simulink model "poredjenje_regulatora_nelinearni_model"  (R2018a)
settings: Solver=ode4  StartTime=0.0  StopTime=150  FixedStep=0.01  RelTol=1e-3  EnableMultiTasking=on
values from neighbouring files (symbols this model uses):
  a1 = K_dek(1, 1)    [skript_drugi_deo.m]
  a2 = K_dek(1, 2)    [skript_drugi_deo.m]
  a3 = K_dek(2, 1)    [skript_drugi_deo.m]
  a4 = K_dek(2, 2)    [skript_drugi_deo.m]
  Ar1 = 0.04    [skript_drugi_deo.m]
  Ar2 = 0.04    [skript_drugi_deo.m]
  Cd1 = 0.65    [skript_drugi_deo.m]
  Cd2 = 0.65    [skript_drugi_deo.m]
  Cdh = 0.65    [skript_drugi_deo.m]
  dT = 0.1    [skript_drugi_deo.m]
  g = 9.81    [skript_drugi_deo.m]
  H1_max = 1.5    [skript_drugi_deo.m]
  H1_min = 0    [skript_drugi_deo.m]
  H1_N = 0.7    [skript_drugi_deo.m]
  H2_max = 1.5    [skript_drugi_deo.m]
  H2_min = 0    [skript_drugi_deo.m]
  H2_N = 0.8    [skript_drugi_deo.m]
  Kv1 = 1.5/1000    (= 0.0015)    [skript_drugi_deo.m]
  Kv2 = 1.5/1000    (= 0.0015)    [skript_drugi_deo.m]
  Kvh = 1/1000    (= 0.001)    [skript_drugi_deo.m]
  Ph = 3.25*10^5    (= 325000)    [skript_drugi_deo.m]
  ro = 1000    [skript_drugi_deo.m]
  Uv1 = 3    [skript_drugi_deo.m]
  Uv2_max = 10    [skript_drugi_deo.m]
  Uv2_min = 0    [skript_drugi_deo.m]
  Uv2_N = double(solve(e2 == 0, U2_N))    [skript_drugi_deo.m]
  Uvh_max = 10    [skript_drugi_deo.m]
  Uvh_min = 0    [skript_drugi_deo.m]
  Uvh_N = double(solve(e1 == 0, Uh_N))    [skript_drugi_deo.m]
  w1 = 0.1    [skript_drugi_deo.m]
  w2 = 0.1    [skript_drugi_deo.m]
  wh = 0.03    [skript_drugi_deo.m]
undefined symbols (not defined in the file or in its folder): den_d1, den_d2, num_d1, num_d2
libraries: simulink x2
settings Model: Creator=Nikola  LastModifiedBy=lakim
settings DataIOCC: LimitDataPoints=on  SaveFormat=Array
settings OptimizationCC: LifeSpan=inf
settings DebuggingCC: SFUnexpectedBacktrackingDiag=warning  SFNoUnconditionalDefaultTransitionDiag=warning  SFExecutionAtInitializationDiag=none
settings HardwareCC: ProdBitPerPointer=32  ProdBitPerSizeT=32  ProdBitPerPtrDiffT=32  ProdLargestAtomicFloat=None  ProdIntDivRoundTo=Undefined  ProdEndianess=Unspecified  ProdWordSize=32  ProdHWDeviceType=32-bit Generic
settings ModelReferenceCC: PropagateSignalLabelsOutOfModel=off
settings CodeAppCC: StateflowObjectComments=on
settings GRTTargetCC: TargetLangStandard=C89/C90 (ANSI)  GeneratePreprocessorConditionals=Disable all
settings ConfigComp: CovMetricSettings=dw  CovHtmlReporting=on  CovSaveCumulativeToWorkspaceVar=on  CovSaveSingleToWorkspaceVar=on  CovExternalEMLEnable=off

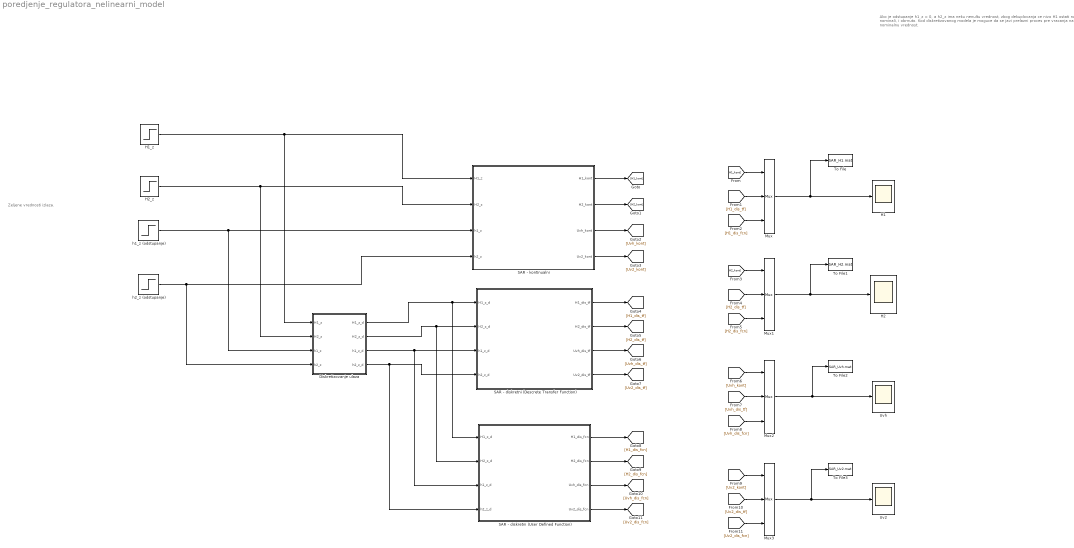
== system poredjenje_regulatora_nelinearni_model ==
  note: Ako je odstupanje h1_z = 0, a h2_z ima neku nenultu vrednost,
      | zbog dekuplovanja ce nivo H1 ostati na nominali, i obrnuto.
      | Kod diskretizovanog modela je moguce da se javi prelazni
      | proces pre vracanja na nominalnu vrednost.
  note: Zeljene vrednosti izlaza.
  Diskretizovanje ulaza : Subsystem
  H1 : Scope
  "H1_z " : Step  Time=0  After=H1_N  SampleTime=0
  H2 : Scope
  H2_z : Step  Time=0  After=H2_N  SampleTime=0
  Mux{,1..3} (4 alike) : Mux  Inputs=3
  SAR - diskretni (Descrete Transfer Function) : Subsystem
  SAR - diskretni (User Defined Function) : Subsystem
  SAR - kontinualni : Subsystem
  To File : ToFile  Filename=SAR_H1.mat  MatrixName=H1_r
  To File1 : ToFile  Filename=SAR_H2.mat  MatrixName=H2_r
  To File2 : ToFile  Filename=SAR_Uvh.mat  MatrixName=Uvh_r
  To File3 : ToFile  Filename=SAR_Uv2.mat  MatrixName=Uv2_r
  "Uv2 " : Scope
  "Uvh  " : Scope
  h1_z (odstupanje) : Step  Time=0  After=0.1  SampleTime=0
  h2_z (odstupanje) : Step  Time=0  After=0  SampleTime=0
  wires:
  "H1_z "/1 -> Diskretizovanje ulaza/1(H1_z), SAR - kontinualni/1(H1_z)
  H2_z/1 -> Diskretizovanje ulaza/2(H2_z), SAR - kontinualni/2(H2_z)
  h1_z (odstupanje)/1 -> Diskretizovanje ulaza/3(h1_z), SAR - kontinualni/3(h1_z)
  h2_z (odstupanje)/1 -> Diskretizovanje ulaza/4(h2_z), SAR - kontinualni/4(h2_z)
  Diskretizovanje ulaza/1(H1_z_d) -> SAR - diskretni (User Defined Function)/1(H1_z_d), SAR - diskretni (Descrete Transfer Function)/1(H1_z_d)
  Diskretizovanje ulaza/2(H2_z_d) -> SAR - diskretni (User Defined Function)/2(H2_z_d), SAR - diskretni (Descrete Transfer Function)/2(H2_z_d)
  Diskretizovanje ulaza/3(h1_z_d) -> SAR - diskretni (User Defined Function)/3(h1_z_d), SAR - diskretni (Descrete Transfer Function)/3(h1_z_d)
  Diskretizovanje ulaza/4(h2_z_d) -> SAR - diskretni (User Defined Function)/4(h2_z_d), SAR - diskretni (Descrete Transfer Function)/4(h2_z_d)
  Mux/1 -> To File/1, H1/1
  Mux1/1 -> To File1/1, H2/1
  SAR - kontinualni/1(H1_kont) -> [H1_kont]
  SAR - kontinualni/2(H2_kont) -> [H2_kont]
  SAR - kontinualni/3(Uvh_kont) -> [Uvh_kont]
  SAR - kontinualni/4(Uv2_kont) -> [Uv2_kont]
  SAR - diskretni (Descrete Transfer Function)/1(H1_dis_tf) -> [H1_dis_tf]
  SAR - diskretni (Descrete Transfer Function)/2(H2_dis_tf) -> [H2_dis_tf]
  SAR - diskretni (Descrete Transfer Function)/3(Uvh_dis_tf) -> [Uvh_dis_tf]
  SAR - diskretni (Descrete Transfer Function)/4(Uv2_dis_tf) -> [Uv2_dis_tf]
  [H2_kont] -> Mux1/1
  [H2_dis_tf] -> Mux1/2
  [H2_dis_fcn] -> Mux1/3
  [Uvh_dis_tf] -> Mux2/2
  [Uvh_kont] -> Mux2/1
  [Uvh_dis_fcn] -> Mux2/3
  [Uv2_kont] -> Mux3/1
  [Uv2_dis_tf] -> Mux3/2
  [Uv2_dis_fcn] -> Mux3/3
  Mux2/1 -> To File2/1, "Uvh  "/1
  Mux3/1 -> To File3/1, "Uv2 "/1
  [H1_kont] -> Mux/1
  [H1_dis_tf] -> Mux/2
  [H1_dis_fcn] -> Mux/3
  SAR - diskretni (User Defined Function)/1(H1_dis_fcn) -> [H1_dis_fcn]
  SAR - diskretni (User Defined Function)/2(H2_dis_fcn) -> [H2_dis_fcn]
  SAR - diskretni (User Defined Function)/3(Uvh_dis_fcn) -> [Uvh_dis_fcn]
  SAR - diskretni (User Defined Function)/4(Uv2_dis_fcn) -> [Uv2_dis_fcn]

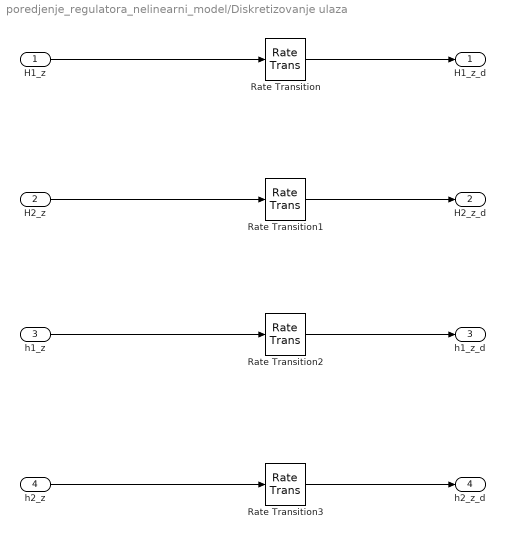
== system poredjenje_regulatora_nelinearni_model/Diskretizovanje ulaza ==
  H1_z : Inport
  H2_z : Inport  Port=2
  h1_z : Inport  Port=3
  h2_z : Inport  Port=4
  Rate Transition : RateTransition  OutPortSampleTime=dT
  Rate Transition1 : RateTransition  OutPortSampleTime=dT
  Rate Transition2 : RateTransition  OutPortSampleTime=dT
  Rate Transition3 : RateTransition  InitialCondition=dT
  H1_z_d : Outport
  H2_z_d : Outport  Port=2
  h1_z_d : Outport  Port=3
  h2_z_d : Outport  Port=4
  wires:
  H1_z/1 -> Rate Transition/1
  Rate Transition/1 -> H1_z_d/1
  H2_z/1 -> Rate Transition1/1
  Rate Transition1/1 -> H2_z_d/1
  h1_z/1 -> Rate Transition2/1
  Rate Transition2/1 -> h1_z_d/1
  h2_z/1 -> Rate Transition3/1
  Rate Transition3/1 -> h2_z_d/1

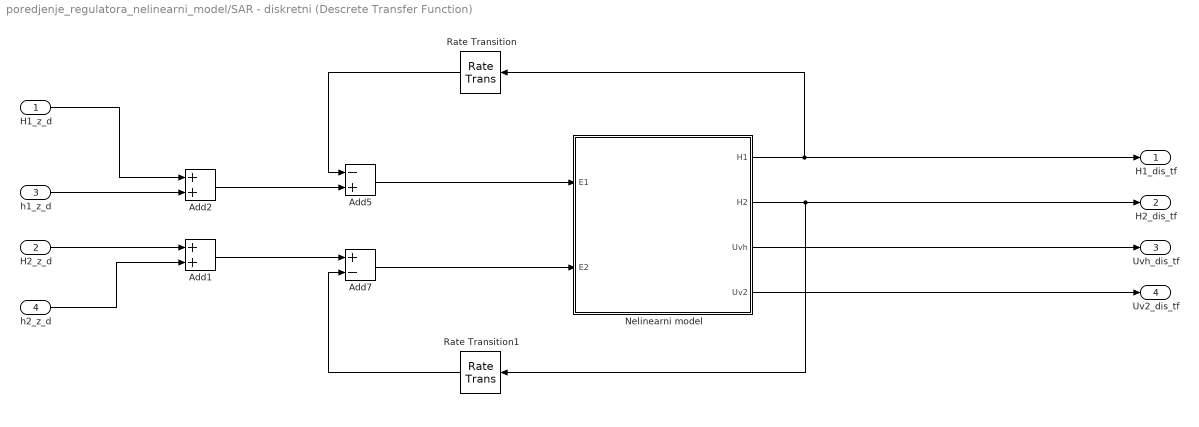
== system poredjenje_regulatora_nelinearni_model/SAR - diskretni (Descrete Transfer Function) ==
  H1_z_d : Inport
  H2_z_d : Inport  Port=2
  h1_z_d : Inport  Port=3
  h2_z_d : Inport  Port=4
  Add1 : Sum
  Add2 : Sum
  Add5 : Sum  Inputs=-+
  Add7 : Sum  Inputs=+-
  "Nelinearni model " : Subsystem
  Rate Transition : RateTransition  OutPortSampleTime=dT
  Rate Transition1 : RateTransition  OutPortSampleTime=dT
  H1_dis_tf : Outport
  H2_dis_tf : Outport  Port=2
  Uvh_dis_tf : Outport  Port=3
  Uv2_dis_tf : Outport  Port=4
  wires:
  "Nelinearni model "/1(H1) -> H1_dis_tf/1, Rate Transition/1
  "Nelinearni model "/2(H2) -> H2_dis_tf/1, Rate Transition1/1
  Add2/1 -> Add5/2
  Add5/1 -> "Nelinearni model "/1(E1)
  Add7/1 -> "Nelinearni model "/2(E2)
  Add1/1 -> Add7/1
  H1_z_d/1 -> Add2/1
  H2_z_d/1 -> Add1/1
  h1_z_d/1 -> Add2/2
  h2_z_d/1 -> Add1/2
  "Nelinearni model "/3(Uvh) -> Uvh_dis_tf/1
  "Nelinearni model "/4(Uv2) -> Uv2_dis_tf/1
  Rate Transition/1 -> Add5/1
  Rate Transition1/1 -> Add7/2

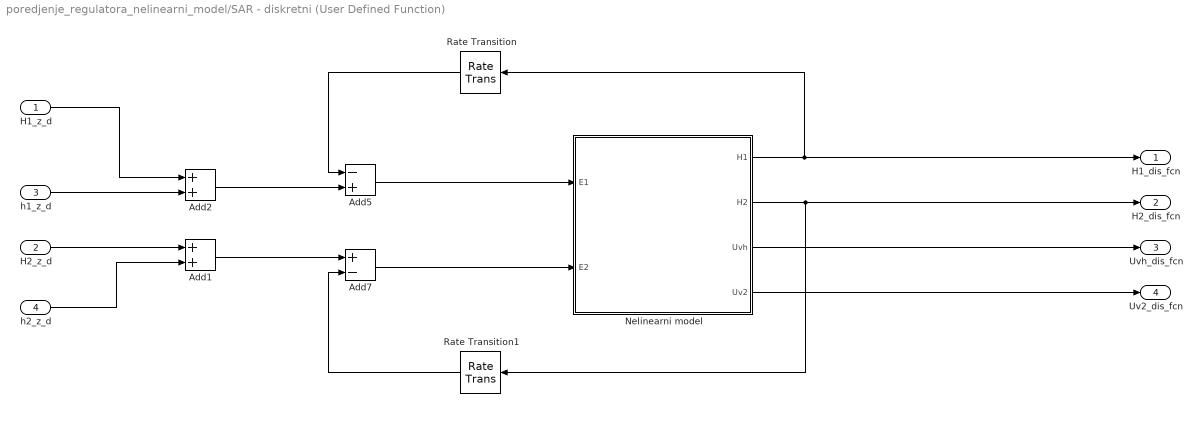
== system poredjenje_regulatora_nelinearni_model/SAR - diskretni (User Defined Function) ==
  H1_z_d : Inport
  H2_z_d : Inport  Port=2
  h1_z_d : Inport  Port=3
  h2_z_d : Inport  Port=4
  Add1 : Sum
  Add2 : Sum
  Add5 : Sum  Inputs=-+
  Add7 : Sum  Inputs=+-
  "Nelinearni model " : Subsystem
  Rate Transition : RateTransition  OutPortSampleTime=dT
  Rate Transition1 : RateTransition  OutPortSampleTime=dT
  H1_dis_fcn : Outport
  H2_dis_fcn : Outport  Port=2
  Uvh_dis_fcn : Outport  Port=3
  Uv2_dis_fcn : Outport  Port=4
  wires:
  "Nelinearni model "/1(H1) -> H1_dis_fcn/1, Rate Transition/1
  "Nelinearni model "/2(H2) -> H2_dis_fcn/1, Rate Transition1/1
  Add2/1 -> Add5/2
  Add5/1 -> "Nelinearni model "/1(E1)
  Add7/1 -> "Nelinearni model "/2(E2)
  Add1/1 -> Add7/1
  H1_z_d/1 -> Add2/1
  H2_z_d/1 -> Add1/1
  h1_z_d/1 -> Add2/2
  h2_z_d/1 -> Add1/2
  "Nelinearni model "/3(Uvh) -> Uvh_dis_fcn/1
  "Nelinearni model "/4(Uv2) -> Uv2_dis_fcn/1
  Rate Transition/1 -> Add5/1
  Rate Transition1/1 -> Add7/2

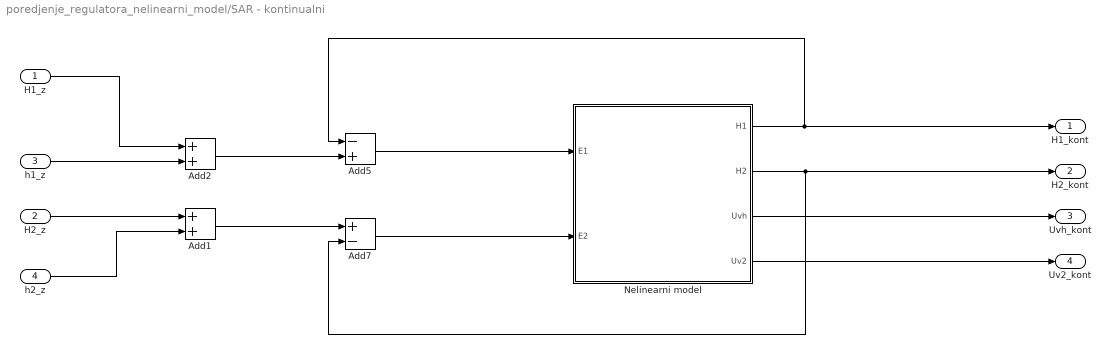
== system poredjenje_regulatora_nelinearni_model/SAR - kontinualni ==
  H1_z : Inport
  H2_z : Inport  Port=2
  h1_z : Inport  Port=3
  h2_z : Inport  Port=4
  Add1 : Sum
  Add2 : Sum
  Add5 : Sum  Inputs=-+
  Add7 : Sum  Inputs=+-
  "Nelinearni model " : Subsystem
  H1_kont : Outport
  H2_kont : Outport  Port=2
  Uvh_kont : Outport  Port=3
  Uv2_kont : Outport  Port=4
  wires:
  "Nelinearni model "/1(H1) -> H1_kont/1, Add5/1
  "Nelinearni model "/2(H2) -> H2_kont/1, Add7/2
  Add2/1 -> Add5/2
  Add5/1 -> "Nelinearni model "/1(E1)
  Add7/1 -> "Nelinearni model "/2(E2)
  Add1/1 -> Add7/1
  H1_z/1 -> Add2/1
  H2_z/1 -> Add1/1
  h1_z/1 -> Add2/2
  h2_z/1 -> Add1/2
  "Nelinearni model "/3(Uvh) -> Uvh_kont/1
  "Nelinearni model "/4(Uv2) -> Uv2_kont/1

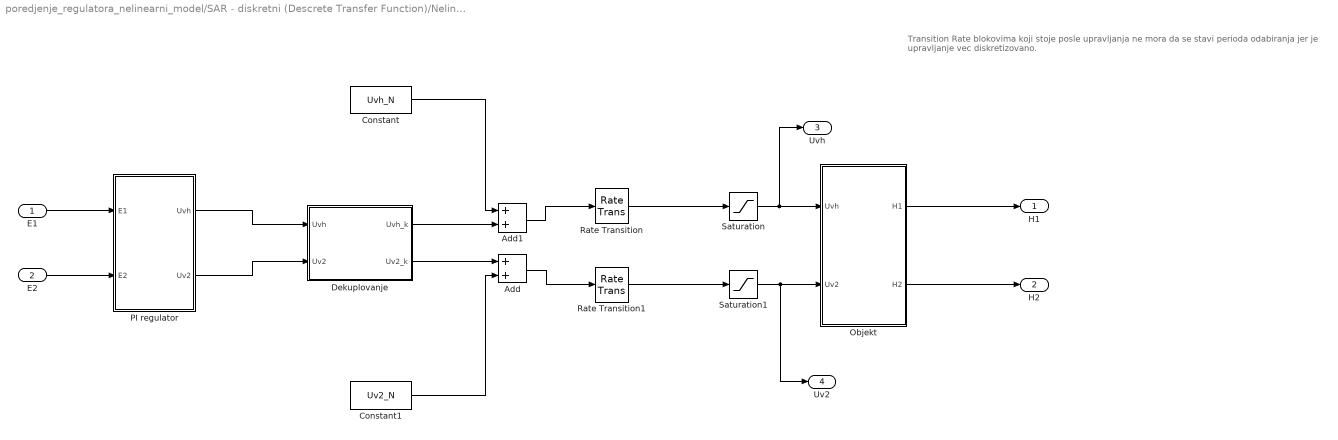
== system poredjenje_regulatora_nelinearni_model/SAR - diskretni (Descrete Transfer Function)/Nelinearni model  ==
  note: Transition Rate blokovima koji stoje posle upravljanja
      | ne mora da se stavi perioda odabiranja jer je upravljanje vec diskretizovano.
  E1 : Inport
  E2 : Inport  Port=2
  Add : Sum
  Add1 : Sum
  Constant : Constant  Value=Uvh_N
  Constant1 : Constant  Value=Uv2_N
  Dekuplovanje : Subsystem
  Objekt : Subsystem
  PI regulator : Subsystem
  Rate Transition : RateTransition
  Rate Transition1 : RateTransition
  Saturation : Saturate  UpperLimit=Uvh_max  LowerLimit=Uvh_min
  Saturation1 : Saturate  UpperLimit=Uv2_max  LowerLimit=Uv2_min
  H1 : Outport
  H2 : Outport  Port=2
  Uvh : Outport  Port=3
  Uv2 : Outport  Port=4
  wires:
  Objekt/1(H1) -> H1/1
  Objekt/2(H2) -> H2/1
  E2/1 -> PI regulator/2(E2)
  E1/1 -> PI regulator/1(E1)
  Saturation/1 -> Uvh/1, Objekt/1(Uvh)
  Saturation1/1 -> Uv2/1, Objekt/2(Uv2)
  Add1/1 -> Rate Transition/1
  Add/1 -> Rate Transition1/1
  Constant1/1 -> Add/2
  Constant/1 -> Add1/1
  Dekuplovanje/1(Uvh_k) -> Add1/2
  Dekuplovanje/2(Uv2_k) -> Add/1
  PI regulator/1(Uvh) -> Dekuplovanje/1(Uvh)
  PI regulator/2(Uv2) -> Dekuplovanje/2(Uv2)
  Rate Transition/1 -> Saturation/1
  Rate Transition1/1 -> Saturation1/1

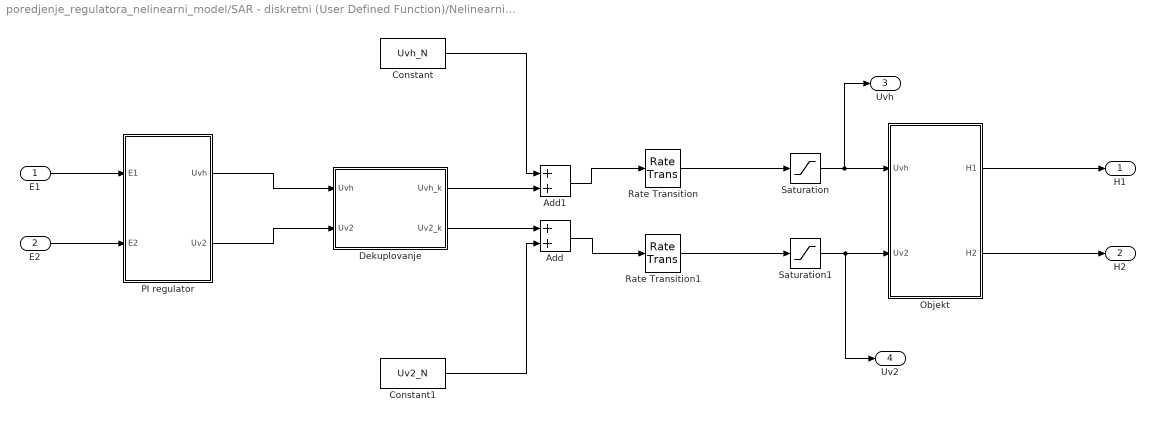
== system poredjenje_regulatora_nelinearni_model/SAR - diskretni (User Defined Function)/Nelinearni model  ==
  E1 : Inport
  E2 : Inport  Port=2
  Add : Sum
  Add1 : Sum
  Constant : Constant  Value=Uvh_N
  Constant1 : Constant  Value=Uv2_N
  Dekuplovanje : Subsystem
  Objekt : Subsystem
  PI regulator : Subsystem
  Rate Transition : RateTransition
  Rate Transition1 : RateTransition
  Saturation : Saturate  UpperLimit=Uvh_max  LowerLimit=Uvh_min
  Saturation1 : Saturate  UpperLimit=Uv2_max  LowerLimit=Uv2_min
  H1 : Outport
  H2 : Outport  Port=2
  Uvh : Outport  Port=3
  Uv2 : Outport  Port=4
  wires:
  Objekt/1(H1) -> H1/1
  Objekt/2(H2) -> H2/1
  E2/1 -> PI regulator/2(E2)
  E1/1 -> PI regulator/1(E1)
  Saturation/1 -> Uvh/1, Objekt/1(Uvh)
  Saturation1/1 -> Uv2/1, Objekt/2(Uv2)
  Add1/1 -> Rate Transition/1
  Add/1 -> Rate Transition1/1
  Constant1/1 -> Add/2
  Constant/1 -> Add1/1
  Dekuplovanje/1(Uvh_k) -> Add1/2
  Dekuplovanje/2(Uv2_k) -> Add/1
  PI regulator/1(Uvh) -> Dekuplovanje/1(Uvh)
  PI regulator/2(Uv2) -> Dekuplovanje/2(Uv2)
  Rate Transition/1 -> Saturation/1
  Rate Transition1/1 -> Saturation1/1

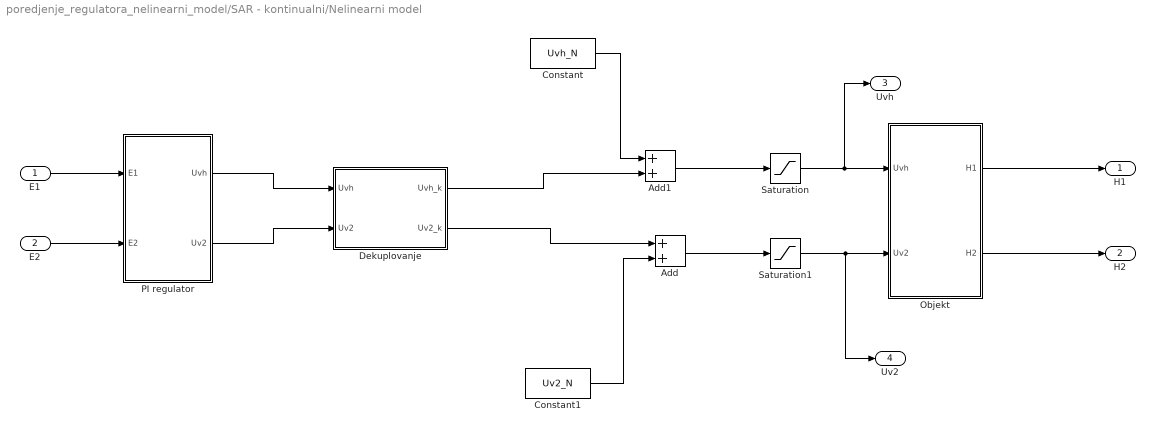
== system poredjenje_regulatora_nelinearni_model/SAR - kontinualni/Nelinearni model  ==
  E1 : Inport
  E2 : Inport  Port=2
  Add : Sum
  Add1 : Sum
  Constant : Constant  Value=Uvh_N
  Constant1 : Constant  Value=Uv2_N
  Dekuplovanje : Subsystem
  Objekt : Subsystem
  PI regulator : Subsystem
  Saturation : Saturate  UpperLimit=Uvh_max  LowerLimit=Uvh_min
  Saturation1 : Saturate  UpperLimit=Uv2_max  LowerLimit=Uv2_min
  H1 : Outport
  H2 : Outport  Port=2
  Uvh : Outport  Port=3
  Uv2 : Outport  Port=4
  wires:
  Objekt/1(H1) -> H1/1
  Objekt/2(H2) -> H2/1
  E2/1 -> PI regulator/2(E2)
  E1/1 -> PI regulator/1(E1)
  Saturation/1 -> Uvh/1, Objekt/1(Uvh)
  Saturation1/1 -> Uv2/1, Objekt/2(Uv2)
  Add1/1 -> Saturation/1
  Add/1 -> Saturation1/1
  Constant1/1 -> Add/2
  Constant/1 -> Add1/1
  Dekuplovanje/1(Uvh_k) -> Add1/2
  Dekuplovanje/2(Uv2_k) -> Add/1
  PI regulator/1(Uvh) -> Dekuplovanje/1(Uvh)
  PI regulator/2(Uv2) -> Dekuplovanje/2(Uv2)

== system poredjenje_regulatora_nelinearni_model/SAR - diskretni (Descrete Transfer Function)/Nelinearni model /Dekuplovanje ==
  Uvh : Inport
  Uv2 : Inport  Port=2
  Add : Sum
  Add1 : Sum
  Gain : Gain  Gain=a1
  Gain1 : Gain  Gain=a2
  Gain2 : Gain  Gain=a3
  Gain3 : Gain  Gain=a4
  Uvh_k : Outport
  Uv2_k : Outport  Port=2
  wires:
  Uvh/1 -> Gain2/1, Gain/1
  Uv2/1 -> Gain1/1, Gain3/1
  Gain/1 -> Add/1
  Gain1/1 -> Add/2
  Gain2/1 -> Add1/1
  Gain3/1 -> Add1/2
  Add/1 -> Uvh_k/1
  Add1/1 -> Uv2_k/1

== system poredjenje_regulatora_nelinearni_model/SAR - diskretni (Descrete Transfer Function)/Nelinearni model /Objekt ==
  Uvh : Inport
  Uv2 : Inport  Port=2
  Jednacina kontionuiteta za rezervoar 1 : Subsystem
  Jednacina kontionuiteta za rezervoar 2 : Subsystem
  H1 : Outport
  H2 : Outport  Port=2
  wires:
  Jednacina kontionuiteta za rezervoar 1/1(H1) -> [H1], H1/1
  Uvh/1 -> Jednacina kontionuiteta za rezervoar 1/1(Uvh)
  Uv2/1 -> Jednacina kontionuiteta za rezervoar 2/2(Uv2)
  Jednacina kontionuiteta za rezervoar 2/1(H2) -> H2/1
  [H1] -> Jednacina kontionuiteta za rezervoar 2/1(H1)

== system poredjenje_regulatora_nelinearni_model/SAR - diskretni (Descrete Transfer Function)/Nelinearni model /PI regulator ==
  E1 : Inport
  E2 : Inport  Port=2
  Discrete Transfer Fcn : DiscreteTransferFcn  Numerator=[num_d1]  Denominator=[den_d1]  SampleTime=dT
  Discrete Transfer Fcn1 : DiscreteTransferFcn  Numerator=[num_d2]  Denominator=[den_d2]  SampleTime=dT
  Uvh : Outport
  Uv2 : Outport  Port=2
  wires:
  E2/1 -> Discrete Transfer Fcn1/1
  E1/1 -> Discrete Transfer Fcn/1
  Discrete Transfer Fcn/1 -> Uvh/1
  Discrete Transfer Fcn1/1 -> Uv2/1

== system poredjenje_regulatora_nelinearni_model/SAR - diskretni (User Defined Function)/Nelinearni model /Dekuplovanje ==
  Uvh : Inport
  Uv2 : Inport  Port=2
  Add : Sum
  Add1 : Sum
  Gain : Gain  Gain=a1
  Gain1 : Gain  Gain=a2
  Gain2 : Gain  Gain=a3
  Gain3 : Gain  Gain=a4
  Uvh_k : Outport
  Uv2_k : Outport  Port=2
  wires:
  Uvh/1 -> Gain2/1, Gain/1
  Uv2/1 -> Gain1/1, Gain3/1
  Gain/1 -> Add/1
  Gain1/1 -> Add/2
  Gain2/1 -> Add1/1
  Gain3/1 -> Add1/2
  Add/1 -> Uvh_k/1
  Add1/1 -> Uv2_k/1

== system poredjenje_regulatora_nelinearni_model/SAR - diskretni (User Defined Function)/Nelinearni model /Objekt ==
  Uvh : Inport
  Uv2 : Inport  Port=2
  Jednacina kontionuiteta za rezervoar 1 : Subsystem
  Jednacina kontionuiteta za rezervoar 2 : Subsystem
  H1 : Outport
  H2 : Outport  Port=2
  wires:
  Jednacina kontionuiteta za rezervoar 1/1(H1) -> [H1], H1/1
  Uvh/1 -> Jednacina kontionuiteta za rezervoar 1/1(Uvh)
  Uv2/1 -> Jednacina kontionuiteta za rezervoar 2/2(Uv2)
  Jednacina kontionuiteta za rezervoar 2/1(H2) -> H2/1
  [H1] -> Jednacina kontionuiteta za rezervoar 2/1(H1)

== system poredjenje_regulatora_nelinearni_model/SAR - diskretni (User Defined Function)/Nelinearni model /PI regulator ==
  note: Korisnicka funkcija daje diferencne jednacine, koje se mogu i dobiti
      | iz diskretne prenosne funkcije, pa su to samim tim dve potpuno analogne stvari.
  E1 : Inport
  E2 : Inport  Port=2
  MATLAB Function : MATLAB Function  TreatAsAtomicUnit=on
  MATLAB Function1 : MATLAB Function  TreatAsAtomicUnit=on
  Uvh : Outport
  Uv2 : Outport  Port=2
  wires:
  E1/1 -> MATLAB Function/1(ek)
  MATLAB Function/1(uk) -> Uvh/1
  E2/1 -> MATLAB Function1/1(ek)
  MATLAB Function1/1(uk) -> Uv2/1

== system poredjenje_regulatora_nelinearni_model/SAR - kontinualni/Nelinearni model /Dekuplovanje ==
  Uvh : Inport
  Uv2 : Inport  Port=2
  Add : Sum
  Add1 : Sum
  Gain : Gain  Gain=a1
  Gain1 : Gain  Gain=a2
  Gain2 : Gain  Gain=a3
  Gain3 : Gain  Gain=a4
  Uvh_k : Outport
  Uv2_k : Outport  Port=2
  wires:
  Uvh/1 -> Gain2/1, Gain/1
  Uv2/1 -> Gain1/1, Gain3/1
  Gain/1 -> Add/1
  Gain1/1 -> Add/2
  Gain2/1 -> Add1/1
  Gain3/1 -> Add1/2
  Add/1 -> Uvh_k/1
  Add1/1 -> Uv2_k/1

== system poredjenje_regulatora_nelinearni_model/SAR - kontinualni/Nelinearni model /Objekt ==
  Uvh : Inport
  Uv2 : Inport  Port=2
  Jednacina kontionuiteta za rezervoar 1 : Subsystem
  Jednacina kontionuiteta za rezervoar 2 : Subsystem
  H1 : Outport
  H2 : Outport  Port=2
  wires:
  Jednacina kontionuiteta za rezervoar 1/1(H1) -> [H1], H1/1
  Uvh/1 -> Jednacina kontionuiteta za rezervoar 1/1(Uvh)
  Uv2/1 -> Jednacina kontionuiteta za rezervoar 2/2(Uv2)
  Jednacina kontionuiteta za rezervoar 2/1(H2) -> H2/1
  [H1] -> Jednacina kontionuiteta za rezervoar 2/1(H1)

== system poredjenje_regulatora_nelinearni_model/SAR - kontinualni/Nelinearni model /PI regulator ==
  E1 : Inport
  E2 : Inport  Port=2
  PID Controller : simulink/Continuous/PID Controller  Controller=PI  TimeDomain=Continuous-time  SampleTime=-1  IntegratorMethod=Forward Euler  FilterMethod=Forward Euler  Form=Parallel  UseFilter=on  ControllerParametersSource=internal  P=6.58388823392313  I=0.318107260315565  D=0  N=100  InitialConditionSource=internal  InitialConditionForIntegrator=0  InitialConditionForFilter=0  ExternalReset=none  LimitOutput=off  UpperSaturationLimit=inf  LowerSaturationLimit=-inf  LinearizeAsGain=on  AntiWindupMode=none  Kb=1  TrackingMode=off  Kt=1  PParamMin=[]  PParamMax=[]  IParamMin=[]  IParamMax=[]  DParamMin=[]  DParamMax=[]  NParamMin=[]  NParamMax=[]  KbParamMin=[]  KbParamMax=[]  KtParamMin=[]  KtParamMax=[]  POutMin=[]  POutMax=[]  IOutMin=[]  IOutMax=[]  DOutMin=[]  DOutMax=[]  NOutMin=[]  NOutMax=[]  KbOutMin=[]  KbOutMax=[]  KtOutMin=[]  KtOutMax=[]  IntegratorOutMin=[]  IntegratorOutMax=[]  FilterOutMin=[]  FilterOutMax=[]  SumOutMin=[]  SumOutMax=[]  SumI1OutMin=[]  SumI1OutMax=[]  SumI2OutMin=[]  SumI2OutMax=[]  SumI3OutMin=[]  SumI3OutMax=[]  SumDOutMin=[]  SumDOutMax=[]  SaturationOutMin=[]  SaturationOutMax=[]  IntegratorContinuousStateAttributes=''  IntegratorStateMustResolveToSignalObject=off  IntegratorRTWStateStorageClass=Auto  FilterContinuousStateAttributes=''  FilterStateMustResolveToSignalObject=off  FilterRTWStateStorageClass=Auto  DifferentiatorICPrevScaledInput=0  DifferentiatorOutMin=[]  DifferentiatorOutMax=[]  FilterDiffOutCoefMin=[]  FilterDiffOutCoefMax=[]  SumDenOutMin=[]  SumDenOutMax=[]  SumNumOutMin=[]  SumNumOutMax=[]  ReciprocalOutMin=[]  ReciprocalOutMax=[]  DivideOutMin=[]  DivideOutMax=[]  TunerSelectOption=Transfer Function Based (PID Tuner App)
  PID Controller2 : simulink/Continuous/PID Controller  Controller=PI  TimeDomain=Continuous-time  SampleTime=-1  IntegratorMethod=Forward Euler  FilterMethod=Forward Euler  Form=Parallel  UseFilter=on  ControllerParametersSource=internal  P=-9.63504962105945  I=-0.943120785670637  D=0  N=100  InitialConditionSource=internal  InitialConditionForIntegrator=0  InitialConditionForFilter=0  ExternalReset=none  LimitOutput=off  UpperSaturationLimit=inf  LowerSaturationLimit=-inf  LinearizeAsGain=on  AntiWindupMode=none  Kb=1  TrackingMode=off  Kt=1  PParamMin=[]  PParamMax=[]  IParamMin=[]  IParamMax=[]  DParamMin=[]  DParamMax=[]  NParamMin=[]  NParamMax=[]  KbParamMin=[]  KbParamMax=[]  KtParamMin=[]  KtParamMax=[]  POutMin=[]  POutMax=[]  IOutMin=[]  IOutMax=[]  DOutMin=[]  DOutMax=[]  NOutMin=[]  NOutMax=[]  KbOutMin=[]  KbOutMax=[]  KtOutMin=[]  KtOutMax=[]  IntegratorOutMin=[]  IntegratorOutMax=[]  FilterOutMin=[]  FilterOutMax=[]  SumOutMin=[]  SumOutMax=[]  SumI1OutMin=[]  SumI1OutMax=[]  SumI2OutMin=[]  SumI2OutMax=[]  SumI3OutMin=[]  SumI3OutMax=[]  SumDOutMin=[]  SumDOutMax=[]  SaturationOutMin=[]  SaturationOutMax=[]  IntegratorContinuousStateAttributes=''  IntegratorStateMustResolveToSignalObject=off  IntegratorRTWStateStorageClass=Auto  FilterContinuousStateAttributes=''  FilterStateMustResolveToSignalObject=off  FilterRTWStateStorageClass=Auto  DifferentiatorICPrevScaledInput=0  DifferentiatorOutMin=[]  DifferentiatorOutMax=[]  FilterDiffOutCoefMin=[]  FilterDiffOutCoefMax=[]  SumDenOutMin=[]  SumDenOutMax=[]  SumNumOutMin=[]  SumNumOutMax=[]  ReciprocalOutMin=[]  ReciprocalOutMax=[]  DivideOutMin=[]  DivideOutMax=[]  TunerSelectOption=Transfer Function Based (PID Tuner App)
  Uvh : Outport
  Uv2 : Outport  Port=2
  wires:
  E1/1 -> PID Controller/1
  PID Controller/1 -> Uvh/1
  E2/1 -> PID Controller2/1
  PID Controller2/1 -> Uv2/1

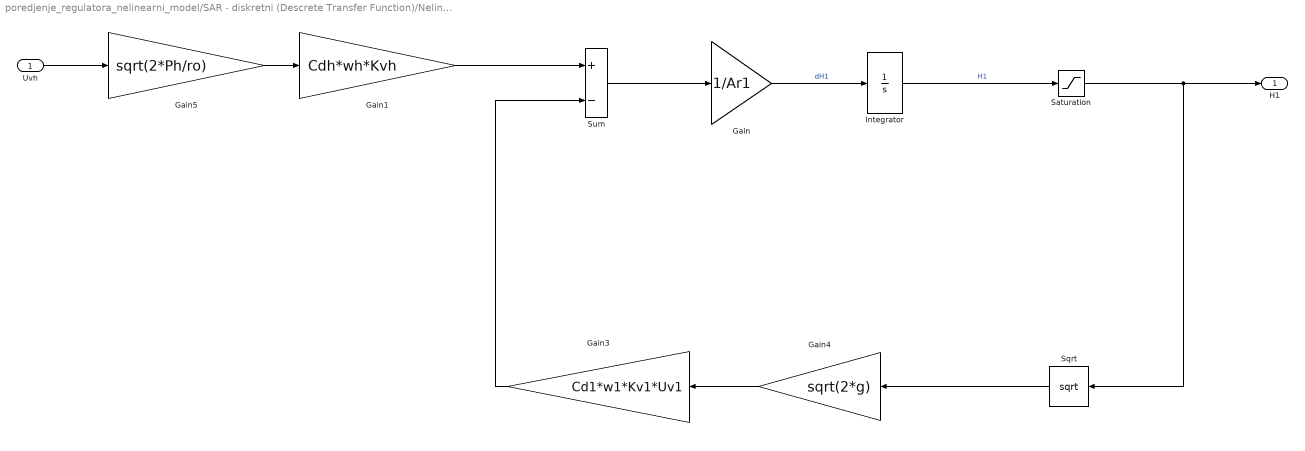
== system poredjenje_regulatora_nelinearni_model/SAR - diskretni (Descrete Transfer Function)/Nelinearni model /Objekt/Jednacina kontionuiteta za rezervoar 1 ==
  Uvh : Inport
  Gain : Gain  Gain=1/Ar1
  Gain1 : Gain  Gain=Cdh*wh*Kvh
  Gain3 : Gain  Gain=Cd1*w1*Kv1*Uv1
  Gain4 : Gain  Gain=sqrt(2*g)
  Gain5 : Gain  Gain=sqrt(2*Ph/ro)
  Integrator : Integrator  InitialCondition=H1_N
  Saturation : Saturate  UpperLimit=H1_max  LowerLimit=H1_min
  Sqrt : Sqrt  SaturateOnIntegerOverflow=on
  Sum : Sum  Inputs=+-
  H1 : Outport
  wires:
  Gain/1 -> Integrator/1  "dH1"
  Sum/1 -> Gain/1
  Integrator/1 -> Saturation/1  "H1"
  Sqrt/1 -> Gain4/1
  Gain4/1 -> Gain3/1
  Gain5/1 -> Gain1/1
  Uvh/1 -> Gain5/1
  Saturation/1 -> Sqrt/1, H1/1
  Gain3/1 -> Sum/2
  Gain1/1 -> Sum/1

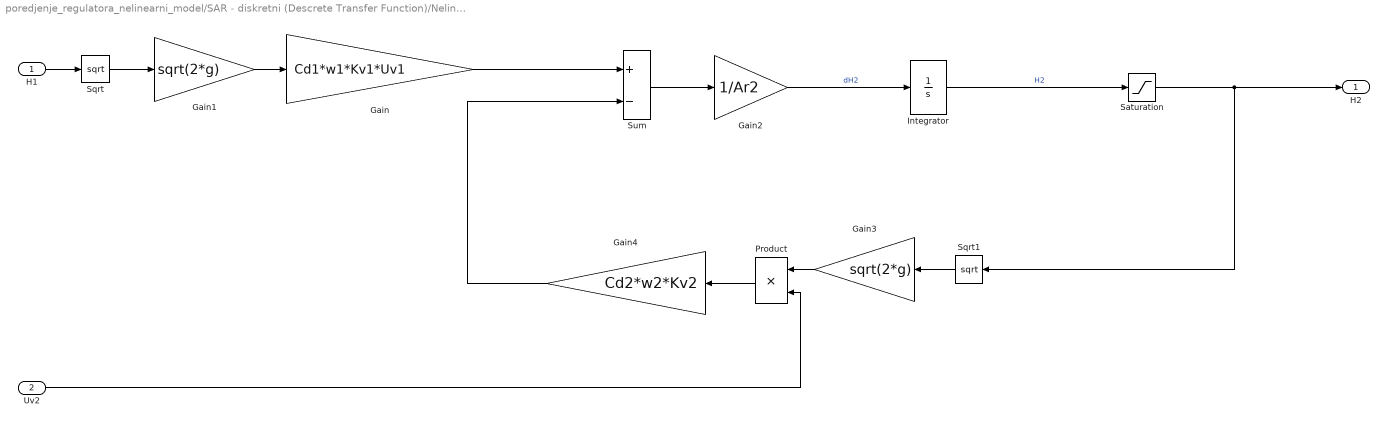
== system poredjenje_regulatora_nelinearni_model/SAR - diskretni (Descrete Transfer Function)/Nelinearni model /Objekt/Jednacina kontionuiteta za rezervoar 2 ==
  H1 : Inport
  Uv2 : Inport  Port=2
  Gain : Gain  Gain=Cd1*w1*Kv1*Uv1
  Gain1 : Gain  Gain=sqrt(2*g)
  Gain2 : Gain  Gain=1/Ar2
  Gain3 : Gain  Gain=sqrt(2*g)
  Gain4 : Gain  Gain=Cd2*w2*Kv2
  Integrator : Integrator  InitialCondition=H2_N
  Product : Product
  Saturation : Saturate  UpperLimit=H2_max  LowerLimit=H2_min
  Sqrt : Sqrt  SaturateOnIntegerOverflow=on
  Sqrt1 : Sqrt  SaturateOnIntegerOverflow=on
  Sum : Sum  Inputs=+-
  H2 : Outport
  wires:
  H1/1 -> Sqrt/1
  Sqrt/1 -> Gain1/1
  Gain1/1 -> Gain/1
  Gain/1 -> Sum/1
  Sum/1 -> Gain2/1
  Gain2/1 -> Integrator/1  "dH2"
  Integrator/1 -> Saturation/1  "H2"
  Sqrt1/1 -> Gain3/1
  Gain3/1 -> Product/1
  Uv2/1 -> Product/2
  Product/1 -> Gain4/1
  Gain4/1 -> Sum/2
  Saturation/1 -> Sqrt1/1, H2/1

== system poredjenje_regulatora_nelinearni_model/SAR - diskretni (User Defined Function)/Nelinearni model /Objekt/Jednacina kontionuiteta za rezervoar 1 ==
  Uvh : Inport
  Gain : Gain  Gain=1/Ar1
  Gain1 : Gain  Gain=Cdh*wh*Kvh
  Gain3 : Gain  Gain=Cd1*w1*Kv1*Uv1
  Gain4 : Gain  Gain=sqrt(2*g)
  Gain5 : Gain  Gain=sqrt(2*Ph/ro)
  Integrator : Integrator  InitialCondition=H1_N
  Saturation : Saturate  UpperLimit=H1_max  LowerLimit=H1_min
  Sqrt : Sqrt  SaturateOnIntegerOverflow=on
  Sum : Sum  Inputs=+-
  H1 : Outport
  wires:
  Gain/1 -> Integrator/1  "dH1"
  Sum/1 -> Gain/1
  Integrator/1 -> Saturation/1  "H1"
  Sqrt/1 -> Gain4/1
  Gain4/1 -> Gain3/1
  Gain5/1 -> Gain1/1
  Uvh/1 -> Gain5/1
  Saturation/1 -> Sqrt/1, H1/1
  Gain3/1 -> Sum/2
  Gain1/1 -> Sum/1

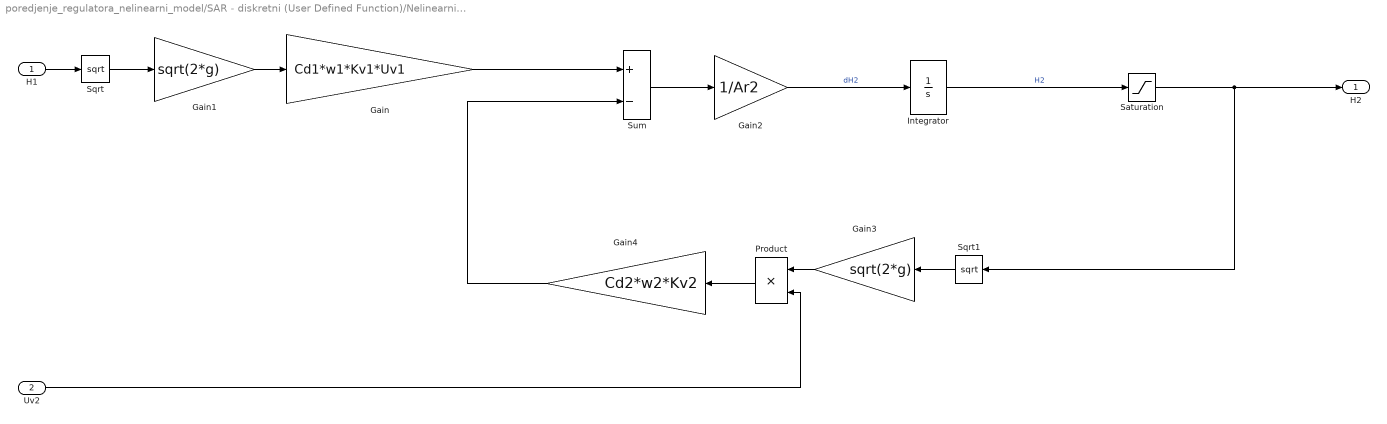
== system poredjenje_regulatora_nelinearni_model/SAR - diskretni (User Defined Function)/Nelinearni model /Objekt/Jednacina kontionuiteta za rezervoar 2 ==
  H1 : Inport
  Uv2 : Inport  Port=2
  Gain : Gain  Gain=Cd1*w1*Kv1*Uv1
  Gain1 : Gain  Gain=sqrt(2*g)
  Gain2 : Gain  Gain=1/Ar2
  Gain3 : Gain  Gain=sqrt(2*g)
  Gain4 : Gain  Gain=Cd2*w2*Kv2
  Integrator : Integrator  InitialCondition=H2_N
  Product : Product
  Saturation : Saturate  UpperLimit=H2_max  LowerLimit=H2_min
  Sqrt : Sqrt  SaturateOnIntegerOverflow=on
  Sqrt1 : Sqrt  SaturateOnIntegerOverflow=on
  Sum : Sum  Inputs=+-
  H2 : Outport
  wires:
  H1/1 -> Sqrt/1
  Sqrt/1 -> Gain1/1
  Gain1/1 -> Gain/1
  Gain/1 -> Sum/1
  Sum/1 -> Gain2/1
  Gain2/1 -> Integrator/1  "dH2"
  Integrator/1 -> Saturation/1  "H2"
  Sqrt1/1 -> Gain3/1
  Gain3/1 -> Product/1
  Uv2/1 -> Product/2
  Product/1 -> Gain4/1
  Gain4/1 -> Sum/2
  Saturation/1 -> Sqrt1/1, H2/1

== system poredjenje_regulatora_nelinearni_model/SAR - kontinualni/Nelinearni model /Objekt/Jednacina kontionuiteta za rezervoar 1 ==
  Uvh : Inport
  Gain : Gain  Gain=1/Ar1
  Gain1 : Gain  Gain=Cdh*wh*Kvh
  Gain3 : Gain  Gain=Cd1*w1*Kv1*Uv1
  Gain4 : Gain  Gain=sqrt(2*g)
  Gain5 : Gain  Gain=sqrt(2*Ph/ro)
  Integrator : Integrator  InitialCondition=H1_N
  Saturation : Saturate  UpperLimit=H1_max  LowerLimit=H1_min
  Sqrt : Sqrt  SaturateOnIntegerOverflow=on
  Sum : Sum  Inputs=+-
  H1 : Outport
  wires:
  Gain/1 -> Integrator/1  "dH1"
  Sum/1 -> Gain/1
  Integrator/1 -> Saturation/1  "H1"
  Sqrt/1 -> Gain4/1
  Gain4/1 -> Gain3/1
  Gain5/1 -> Gain1/1
  Uvh/1 -> Gain5/1
  Saturation/1 -> Sqrt/1, H1/1
  Gain3/1 -> Sum/2
  Gain1/1 -> Sum/1

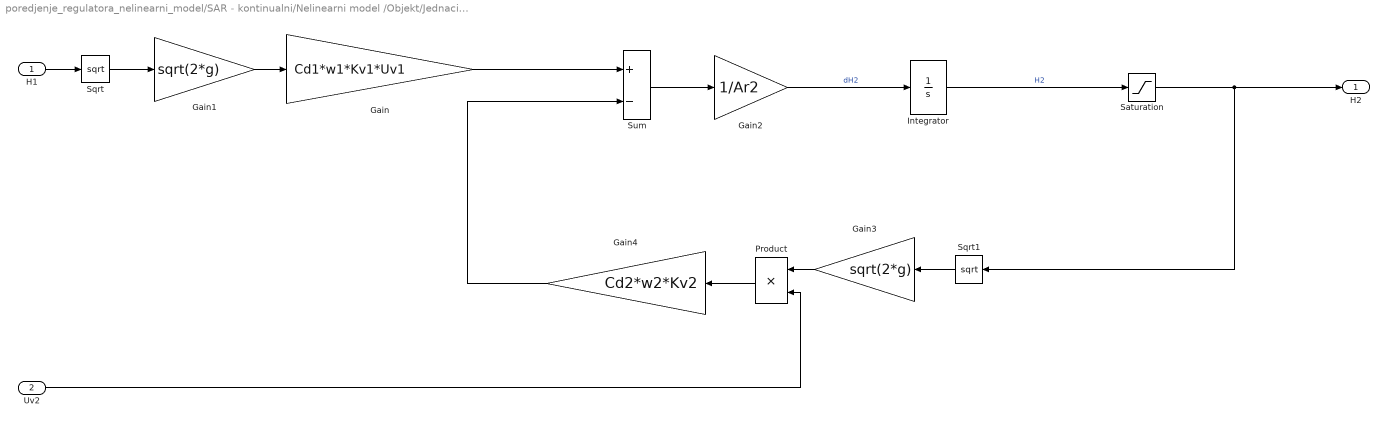
== system poredjenje_regulatora_nelinearni_model/SAR - kontinualni/Nelinearni model /Objekt/Jednacina kontionuiteta za rezervoar 2 ==
  H1 : Inport
  Uv2 : Inport  Port=2
  Gain : Gain  Gain=Cd1*w1*Kv1*Uv1
  Gain1 : Gain  Gain=sqrt(2*g)
  Gain2 : Gain  Gain=1/Ar2
  Gain3 : Gain  Gain=sqrt(2*g)
  Gain4 : Gain  Gain=Cd2*w2*Kv2
  Integrator : Integrator  InitialCondition=H2_N
  Product : Product
  Saturation : Saturate  UpperLimit=H2_max  LowerLimit=H2_min
  Sqrt : Sqrt  SaturateOnIntegerOverflow=on
  Sqrt1 : Sqrt  SaturateOnIntegerOverflow=on
  Sum : Sum  Inputs=+-
  H2 : Outport
  wires:
  H1/1 -> Sqrt/1
  Sqrt/1 -> Gain1/1
  Gain1/1 -> Gain/1
  Gain/1 -> Sum/1
  Sum/1 -> Gain2/1
  Gain2/1 -> Integrator/1  "dH2"
  Integrator/1 -> Saturation/1  "H2"
  Sqrt1/1 -> Gain3/1
  Gain3/1 -> Product/1
  Uv2/1 -> Product/2
  Product/1 -> Gain4/1
  Gain4/1 -> Sum/2
  Saturation/1 -> Sqrt1/1, H2/1

== matlab function poredjenje_regulatora_nelinearni_model/SAR - diskretni (User Defined Function)/Nelinearni model /PI regulator/MATLAB Function1 ==
  data: ek input; uk output
function uk = regulator(ek)

        persistent ek1 uk1 s
        if isempty(s)
            s = 0;
            ek1 = 0;
            uk1 = 0;
        end
        
        b1 = -9.682205660342984;
        b0 = 9.587893581775917;
        a1 = 1;
        a0 = -1;
        uk = 1/a1*(b1*ek + b0*ek1 - a0*uk1);
        uk1 = uk;
        ek1 = ek;

== matlab function poredjenje_regulatora_nelinearni_model/SAR - diskretni (User Defined Function)/Nelinearni model /PI regulator/MATLAB Function ==
  data: ek input; uk output
function uk = regulator(ek)

        persistent ek1 uk1 s
        if isempty(s)
            s = 0;
            ek1 = 0;
            uk1 = 0;
        end
        
        b1 = 6.599793596938907;
        b0 = -6.567982870907351;
        a1 = 1;
        a0 = -1;
        uk = 1/a1*(b1*ek + b0*ek1 - a0*uk1);
        uk1 = uk;
        ek1 = ek;
